simulink subsystem "ControladorReactivo"  (R2023b)
settings: Solver=VariableStepAuto  StartTime=0.0  StopTime=10.0  RelTol=1e-3
settings Model: Creator=Antonio  LastModifiedBy=Antonio

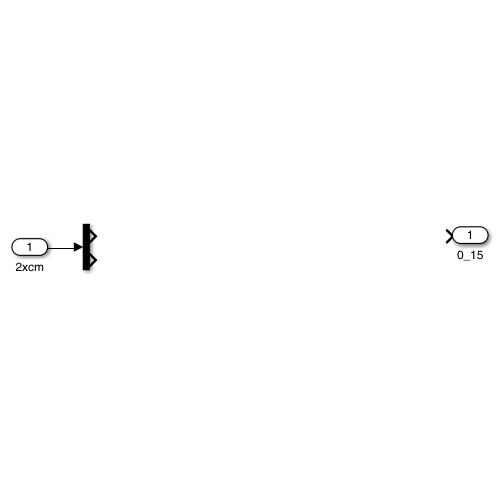
[thumbnail: Simulink's stored preview of the top-level diagram]
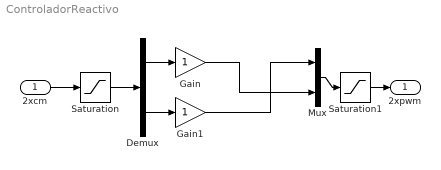
== system ControladorReactivo ==
  2xcm : Inport
  Demux : Demux  Outputs=2
  Gain : Gain
  Gain1 : Gain
  Mux : Mux  Inputs=2
  Saturation : Saturate  UpperLimit=150  LowerLimit=0
  Saturation1 : Saturate  UpperLimit=150  LowerLimit=0
  2xpwm : Outport
  wires:
  2xcm/1 -> Saturation/1
  Mux/1 -> Saturation1/1
  Saturation/1 -> Demux/1
  Demux/1 -> Gain/1
  Demux/2 -> Gain1/1
  Gain/1 -> Mux/2
  Gain1/1 -> Mux/1
  Saturation1/1 -> 2xpwm/1
